simulink model "experiment3_with_12pulse_block"  (R2023a)
settings: Solver=VariableStepAuto  StartTime=0.0  StopTime=0.2  RelTol=1e-3
undefined symbols (not defined in the file): D1, lagging, pulse
libraries: spsUniversalBridgeLib x2, spsCurrentMeasurementLib x1, spsMeanLib x1, spsPLL3phLib x1, spsPulseGeneratorThyristor12PulseLib x1, spsRMSLib x1, spsSeriesRLCBranchLib x1, spsThreePhaseTransformerThreeWindingsLib x1, spsThreePhaseVIMeasurementLib x1, spsThreePhaseSourceLib x1, spsVoltageMeasurementLib x1, sps_lib x1
settings Model: Creator=hp 1  LastModifiedBy=hp 1

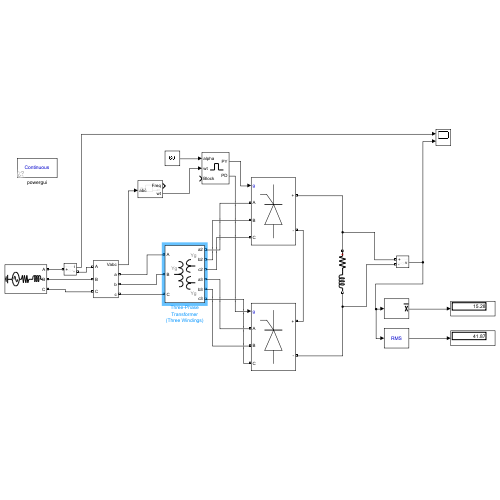
[thumbnail: Simulink's stored preview of the top-level diagram]
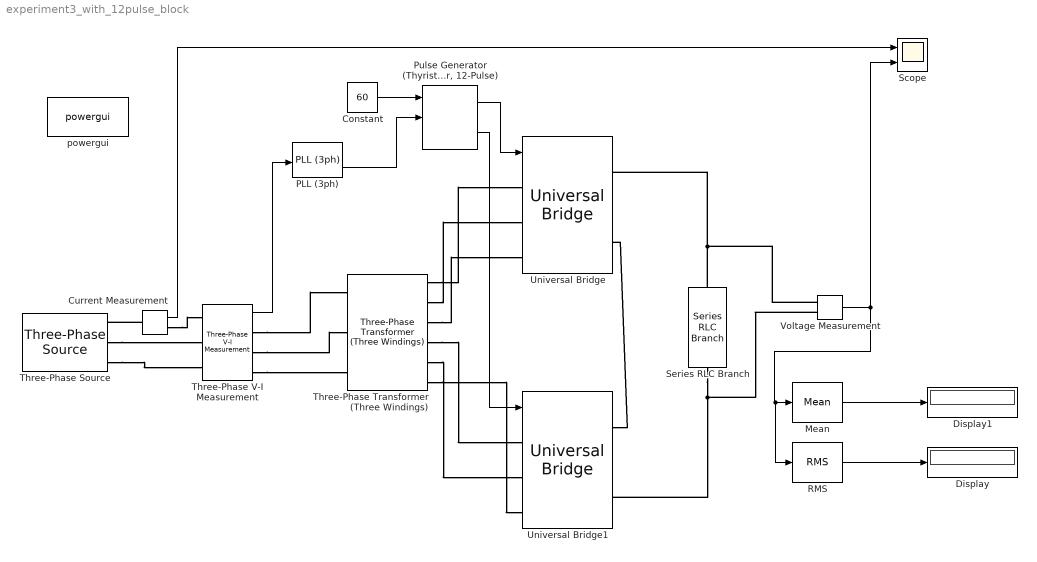
== system experiment3_with_12pulse_block ==
  Constant : Constant  Value=60
  Current Measurement : spsCurrentMeasurementLib/Current Measurement  PhasorSimulation=off  OutputType=Complex  PSBequivalent=0
  Display : Display
  Display1 : Display
  Mean : spsMeanLib/Mean  Freq=50  Vinit=0  Ts=0
  PLL (3ph) : spsPLL3phLib/PLL (3ph)  Fmin=50  Par_Init=[0, 50]  ParK=[180, 3200, 1]  TcD=1e-4  MaxRateChangeFreq=12  FilterCutOffFreq=25  Ts=0  AGC=on
  "Pulse Generator (Thyristor, 12-Pulse)" : spsPulseGeneratorThyristor12PulseLib/Pulse Generator (Thyristor, 12-Pulse)  GenType=12-pulse  Delta=D1 (lagging)  pwidth=60  Double_Pulse=off  Ts=0
      settings: LibrarySourceBlock=|
      | sps_lib/Power Electronics/Power Electronics Control/Pulse Generator
      | (Thyristor, 12-Pulse)
  RMS : spsRMSLib/RMS  TrueRMS=on  Freq=50  RMSInit=120  Ts=0
  Scope : Scope  NumInputPorts=2
  Series RLC Branch : spsSeriesRLCBranchLib/Series RLC Branch  LConnTagsString=__new0  RConnTagsString=__new0  BranchType=RL  Resistance=1  Inductance=10e-3  SetiL0=off  InitialCurrent=0  Capacitance=1e-6  Setx0=off  InitialVoltage=0  Measurements=None
  Three-Phase Transformer (Three Windings) : spsThreePhaseTransformerThreeWindingsLib/Three-Phase Transformer (Three Windings)  Winding1Connection=Yg  Winding2Connection=Yg  Winding3Connection=Yg  CoreType=Three single-phase transformers  SetSaturation=off  Hysteresis=off  DataFile='hysteresis'  SetInitialFlux=off  Measurements=None  UNITS=SI  NominalPower=[ 1000 , 50 ]  Winding1="[320  0 0]"  Winding2=[320 0 0]  Winding3="[320  0 0]"  Rm=1.0804e+06  Lm=2866  L0=0.5  Saturation=[0 0;0.66653 1910.3;277.72 2419.7]  InitialFluxes=[0.8 -0.8 0.7]  BreakLoop=off  DiscreteSolver=Trapezoidal iterative  DataType=on  TransfoNumber=1
      settings: LibrarySourceBlock=|
      | sps_lib/Power Grid Elements/Three-Phase
      | Transformer
      | (Three Windings)
  Three-Phase V-I Measurement : spsThreePhaseVIMeasurementLib/Three-Phase V-I Measurement  VoltageMeasurement=phase-to-ground  SetLabelV=off  LabelV=Vabc  Vpu=off  VpuLL=off  CurrentMeasurement=no  SetLabelI=off  LabelI=Iabc  Ipu=off  Pbase=100e6  Vbase=500e3  OutputType=Complex  PhasorSimulation=off  PSBequivalent=0
  Three-Phase Source : spsThreePhaseSourceLib/Three-Phase Source  InternalConnection=Yg  VoltagePhases=off  Voltage=320  PhaseAngle=0  Voltage_phases=[25e3 25e3 25e3]/sqrt(3)  PhaseAngles_phases=[0 -120 +120]  Frequency=50  NonIdealSource=on  SpecifyImpedance=off  Resistance=0.8929  Inductance=16.58e-3  ShortCircuitLevel=100e6  BaseVoltage=25e3  XRratio=7  BusType=swing  Pref=10e3  Qref=0  Prefabc=[10e3, 10e3, 10e3]  Qrefabc=[0, 0, 0]  Qmin=-inf  Qmax=inf
  Universal Bridge : spsUniversalBridgeLib/Universal Bridge  Arms=3  SnubberResistance=1e5  SnubberCapacitance=inf  Device=Thyristors  Ron=1e-3  Lon=0  ForwardVoltages="[  0  0  ]"  ForwardVoltage=0  GTOparameters=[ 10e-6 , 20e-6 ]  IGBTparameters=[ 1e-6 , 2e-6 ]  Measurements=None  Measurements_2=None  converterType=Rectifier
  Universal Bridge1 : spsUniversalBridgeLib/Universal Bridge  Arms=3  SnubberResistance=1e5  SnubberCapacitance=inf  Device=Thyristors  Ron=1e-3  Lon=0  ForwardVoltages="[  0  0  ]"  ForwardVoltage=0  GTOparameters=[ 10e-6 , 20e-6 ]  IGBTparameters=[ 1e-6 , 2e-6 ]  Measurements=None  Measurements_2=None  converterType=Rectifier
  Voltage Measurement : spsVoltageMeasurementLib/Voltage Measurement  PhasorSimulation=off  OutputType=Complex  PSBequivalent=0
  powergui : sps_lib/powergui  Priority=1  SimulationMode=Continuous  SampleTime=50e-6  frequency=60  Iterations=50  frequencyindice=50  Pbase=100e6  ErrMax=1e-4  UnitsV=kV  UnitsW=MW  buscounter=0  FunctionMessages=off  echomessages=off  EnableUseOfTLC=off  CurrentSourceSwitches=off  DisableSnubberDevices=off  DisableRonSwitches=off  DisableVfSwitches=off  DisplayEquations=off  AutomaticDiscreteSolvers=off  SolverType=Tustin/Backward Euler (TBE)  Interpol=off  ExternalGateDelay=off  methode=off  Ts=100  x0status=blocks  SPID=on  SwTol=0  HookPort=off  NonlinearTolerance=1e-4  nMaxIteration=100  ContinueOnMaxIteration=off  RestoreLinks=warning  ResistiveCurrentMeasurement=off  Frange=[0:2:500]  Ylog=off  Xlog=on  ShowGrid=off  save=off  variable=ZData  structure=0  ZoomFFT=off  StartTime=0.0  cycles=1  DisplayStyle=1  fundamental=60  FreqAxis=off  MaxFrequency=1000  frequencyindicesteady=1  RmsSteady=1  display=off
  wires:
  Current Measurement/1 -> Scope/1
  Three-Phase V-I Measurement/1 -> PLL (3ph)/1
  PLL (3ph)/2 -> "Pulse Generator (Thyristor, 12-Pulse)"/2
  Constant/1 -> "Pulse Generator (Thyristor, 12-Pulse)"/1
  "Pulse Generator (Thyristor, 12-Pulse)"/1 -> Universal Bridge/1
  "Pulse Generator (Thyristor, 12-Pulse)"/2 -> Universal Bridge1/1
  RMS/1 -> Display/1
  Mean/1 -> Display1/1
  Voltage Measurement/1 -> Scope/2, RMS/1, Mean/1
  connections:
  Current Measurement/LConn1 -- Three-Phase Source/RConn1
  Current Measurement/RConn1 -- Three-Phase V-I Measurement/LConn1
  Three-Phase Source/RConn2 -- Three-Phase V-I Measurement/LConn2
  Three-Phase Source/RConn3 -- Three-Phase V-I Measurement/LConn3
  Three-Phase V-I Measurement/RConn1 -- Three-Phase Transformer (Three Windings)/LConn1
  Three-Phase V-I Measurement/RConn2 -- Three-Phase Transformer (Three Windings)/LConn2
  Three-Phase V-I Measurement/RConn3 -- Three-Phase Transformer (Three Windings)/LConn3
  Three-Phase Transformer (Three Windings)/RConn1 -- Universal Bridge/LConn1
  Three-Phase Transformer (Three Windings)/RConn2 -- Universal Bridge/LConn2
  Three-Phase Transformer (Three Windings)/RConn3 -- Universal Bridge/LConn3
  Three-Phase Transformer (Three Windings)/RConn4 -- Universal Bridge1/LConn1
  Three-Phase Transformer (Three Windings)/RConn5 -- Universal Bridge1/LConn2
  Three-Phase Transformer (Three Windings)/RConn6 -- Universal Bridge1/LConn3
  Universal Bridge1/RConn1 -- Universal Bridge/RConn2
  Series RLC Branch/LConn1 -- Voltage Measurement/LConn1 -- Universal Bridge/RConn1
  Series RLC Branch/RConn1 -- Voltage Measurement/LConn2 -- Universal Bridge1/RConn2
